simulink model "bidirectional_LLC"  (R2018a)
settings: Solver=VariableStepDiscrete  StartTime=0.0  StopTime=1  RelTol=1e-3
libraries: powerlib x33
settings Model: Creator=ADHI  LastModifiedBy=ADHI

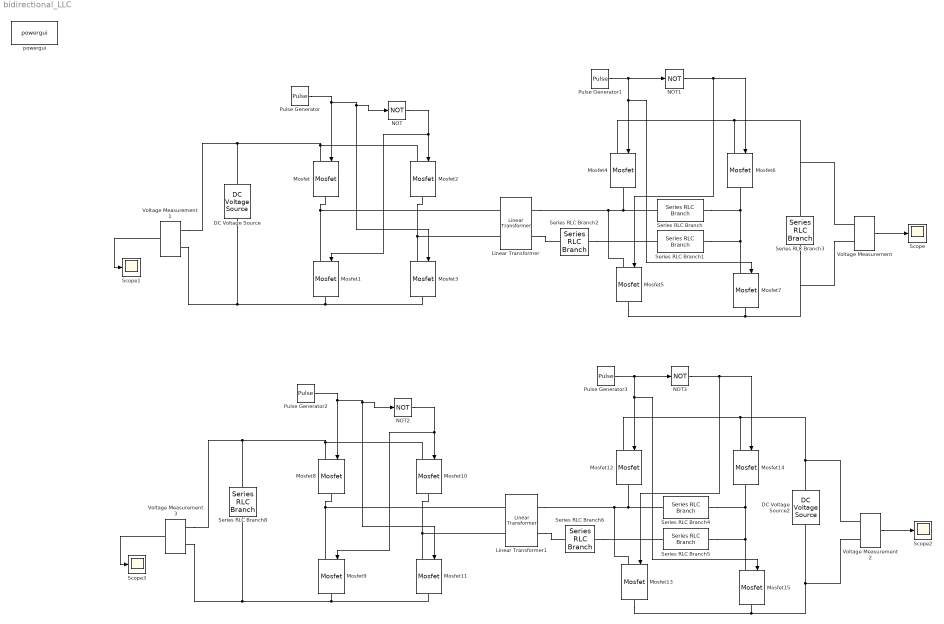
== system bidirectional_LLC ==
  DC Voltage Source : powerlib/Electrical Sources/DC Voltage Source  Amplitude=48  Measurements=None
  DC Voltage Source2 : powerlib/Electrical Sources/DC Voltage Source  Amplitude=12  Measurements=None
  Linear Transformer : powerlib/Elements/Linear Transformer  UNITS=SI  NominalPower=[ 200 85e3 ]  winding1="[52   1e-2  102e-6]"  winding2="[15  1e-2  1.36e-6 ]"  ThreeWindings=off  winding3=[3.15e+05 0.7938 0.084225]  RmLm=[1e4 963e-6]  Measurements=None  DataType=on
  Linear Transformer1 : powerlib/Elements/Linear Transformer  UNITS=SI  NominalPower=[ 260 85e3 ]  winding1="[65   1e-2  102e-6]"  winding2="[15  1e-2  1.36e-6 ]"  ThreeWindings=off  winding3=[3.15e+05 0.7938 0.084225]  RmLm=[1e4 963e-6]  Measurements=None  DataType=on
  Mosfet{,1..15} (16 alike) : powerlib/Power Electronics/Mosfet  Ron=0.1  Lon=0  Rd=0.01  Vfd=0  IC=0  Rs=1e5  Cs=inf  Measurements=off
  NOT{,1..3} (4 alike) : Logic  Operator=NOT  AllPortsSameDT=off  OutDataTypeStr=boolean
  Pulse Generator{,1..3} (4 alike) : DiscretePulseGenerator  PulseType=Time based  Period=1/50000  PulseWidth=25
  Scope{,1..3} (4 alike) : Scope
  Series RLC Branch : powerlib/Elements/Series RLC Branch  LConnTagsString=__new0  RConnTagsString=__new0  BranchType=L  Resistance=1  Inductance=1e-3  SetiL0=off  InitialCurrent=0  Capacitance=1e-6  Setx0=off  InitialVoltage=0  Measurements=None
  Series RLC Branch1 : powerlib/Elements/Series RLC Branch  LConnTagsString=__new0  RConnTagsString=__new0  BranchType=L  Resistance=1  Inductance=1e-5  SetiL0=off  InitialCurrent=0  Capacitance=1e-6  Setx0=off  InitialVoltage=0  Measurements=None
  Series RLC Branch2 : powerlib/Elements/Series RLC Branch  LConnTagsString=__new0  RConnTagsString=__new0  BranchType=C  Resistance=1  Inductance=1e-3  SetiL0=off  InitialCurrent=0  Capacitance=1e-3  Setx0=off  InitialVoltage=0  Measurements=None
  Series RLC Branch3 : powerlib/Elements/Series RLC Branch  LConnTagsString=__new0  RConnTagsString=__new0  BranchType=C  Resistance=1  Inductance=1e-3  SetiL0=off  InitialCurrent=0  Capacitance=0.01  Setx0=off  InitialVoltage=0  Measurements=None
  Series RLC Branch4 : powerlib/Elements/Series RLC Branch  LConnTagsString=__new0  RConnTagsString=__new0  BranchType=L  Resistance=1  Inductance=1e-3  SetiL0=off  InitialCurrent=0  Capacitance=1e-6  Setx0=off  InitialVoltage=0  Measurements=None
  Series RLC Branch5 : powerlib/Elements/Series RLC Branch  LConnTagsString=__new0  RConnTagsString=__new0  BranchType=L  Resistance=1  Inductance=1e-6  SetiL0=off  InitialCurrent=0  Capacitance=1e-6  Setx0=off  InitialVoltage=0  Measurements=None
  Series RLC Branch6 : powerlib/Elements/Series RLC Branch  LConnTagsString=__new0  RConnTagsString=__new0  BranchType=C  Resistance=1  Inductance=1e-3  SetiL0=off  InitialCurrent=0  Capacitance=1e-3  Setx0=off  InitialVoltage=0  Measurements=None
  Series RLC Branch8 : powerlib/Elements/Series RLC Branch  LConnTagsString=__new0  RConnTagsString=__new0  BranchType=C  Resistance=1  Inductance=1e-3  SetiL0=off  InitialCurrent=0  Capacitance=0.01  Setx0=off  InitialVoltage=0  Measurements=None
  Voltage Measurement{,1..3} (4 alike) : powerlib/Measurements/Voltage Measurement  PhasorSimulation=off  OutputType=Complex  PSBequivalent=0
  powergui : powerlib/powergui  Priority=1  SimulationMode=Discrete  SampleTime=50e-6  frequency=60  Iterations=50  frequencyindice=0  Pbase=100e6  ErrMax=1e-4  UnitsV=kV  UnitsW=MW  buscounter=0  FunctionMessages=off  echomessages=off  EnableUseOfTLC=off  CurrentSourceSwitches=off  DisableSnubberDevices=off  DisableRonSwitches=off  DisableVfSwitches=off  DisplayEquations=off  SolverType=Tustin/Backward Euler (TBE)  Interpol=off  ExternalGateDelay=off  methode=off  Ts=100  x0status=blocks  SPID=on  SwTol=0  HookPort=off  RestoreLinks=warning  ResistiveCurrentMeasurement=off  Frange=[0:2:500]  Ylog=off  Xlog=on  ShowGrid=off  save=off  variable=ZData  structure=0  ZoomFFT=off  StartTime=0.0  cycles=1  DisplayStyle=1  fundamental=60  FreqAxis=off  MaxFrequency=1000  frequencyindicesteady=1  RmsSteady=1  display=off
  wires:
  Pulse Generator/1 -> NOT/1, Mosfet3/1, Mosfet/1
  NOT/1 -> Mosfet1/1, Mosfet2/1
  Pulse Generator1/1 -> Mosfet7/1, Mosfet4/1, NOT1/1
  NOT1/1 -> Mosfet5/1, Mosfet6/1
  Voltage Measurement/1 -> Scope/1
  Voltage Measurement1/1 -> Scope1/1
  Voltage Measurement3/1 -> Scope3/1
  Voltage Measurement2/1 -> Scope2/1
  NOT3/1 -> Mosfet14/1, Mosfet13/1
  Pulse Generator3/1 -> NOT3/1, Mosfet12/1, Mosfet15/1
  NOT2/1 -> Mosfet10/1, Mosfet9/1
  Pulse Generator2/1 -> Mosfet8/1, Mosfet11/1, NOT2/1
  connections:
  Mosfet1/LConn1 -- Linear Transformer/LConn1 -- Mosfet/RConn1
  Mosfet3/LConn1 -- Linear Transformer/LConn2 -- Mosfet2/RConn1
  DC Voltage Source/RConn1 -- Voltage Measurement1/LConn1 -- Mosfet2/LConn1 -- Mosfet/LConn1
  DC Voltage Source/LConn1 -- Voltage Measurement1/LConn2 -- Mosfet3/RConn1 -- Mosfet1/RConn1
  Mosfet5/LConn1 -- Series RLC Branch/LConn1 -- Mosfet4/RConn1 -- Linear Transformer/RConn1
  Mosfet7/LConn1 -- Series RLC Branch1/RConn1 -- Series RLC Branch/RConn1 -- Mosfet6/RConn1
  Mosfet4/LConn1 -- Voltage Measurement/LConn1 -- Series RLC Branch3/RConn1 -- Mosfet6/LConn1
  Mosfet5/RConn1 -- Voltage Measurement/LConn2 -- Series RLC Branch3/LConn1 -- Mosfet7/RConn1
  Linear Transformer/RConn2 -- Series RLC Branch2/RConn1
  Series RLC Branch2/LConn1 -- Series RLC Branch1/LConn1
  Linear Transformer1/LConn1 -- Mosfet9/LConn1 -- Mosfet8/RConn1
  Linear Transformer1/LConn2 -- Mosfet10/RConn1 -- Mosfet11/LConn1
  Voltage Measurement3/LConn1 -- Series RLC Branch8/RConn1 -- Mosfet8/LConn1 -- Mosfet10/LConn1
  Voltage Measurement3/LConn2 -- Series RLC Branch8/LConn1 -- Mosfet9/RConn1 -- Mosfet11/RConn1
  Mosfet13/LConn1 -- Linear Transformer1/RConn1 -- Mosfet12/RConn1 -- Series RLC Branch4/LConn1
  Series RLC Branch5/RConn1 -- Mosfet15/LConn1 -- Mosfet14/RConn1 -- Series RLC Branch4/RConn1
  Voltage Measurement2/LConn1 -- DC Voltage Source2/RConn1 -- Mosfet14/LConn1 -- Mosfet12/LConn1
  Voltage Measurement2/LConn2 -- DC Voltage Source2/LConn1 -- Mosfet15/RConn1 -- Mosfet13/RConn1
  Series RLC Branch6/LConn1 -- Series RLC Branch5/LConn1
  Linear Transformer1/RConn2 -- Series RLC Branch6/RConn1
